simulink model "Accelerator_Pedal_Position_Sensor_APP_Coherency"  (R2022b)
settings: Solver=FixedStepDiscrete  StartTime=0.0  StopTime=10.0  RelTol=1e-3
libraries: simulink x5
settings Model: Creator=yasso  LastModifiedBy=yasso
settings DataIOCC: ExternalInput=[tt, u3, u4]  LoadExternalInput=on

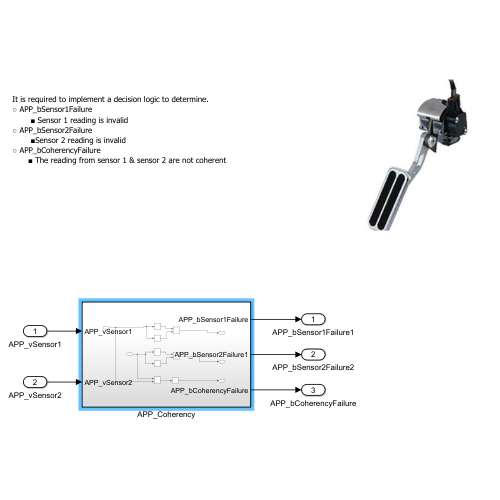
[thumbnail: Simulink's stored preview of the top-level diagram]
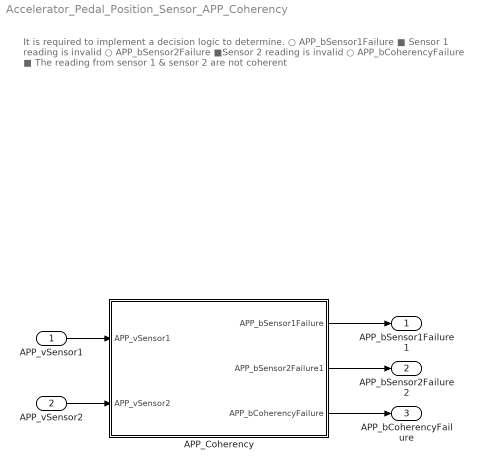
== system Accelerator_Pedal_Position_Sensor_APP_Coherency ==
  note: It is required to implement a decision logic to determine.
      | ○ APP_bSensor1Failure
      | ■ Sensor 1 reading is invalid
      | ○ APP_bSensor2Failure
      | ■Sensor 2 reading is invalid
      | ○ APP_bCoherencyFailure
      | ■ The reading from sensor 1 & sensor 2 are not coherent
  APP_vSensor1 : Inport
  APP_vSensor2 : Inport  Port=2
  APP_Coherency : Subsystem
  APP_bSensor1Failure1 : Outport
  APP_bSensor2Failure2 : Outport  Port=2
  APP_bCoherencyFailure : Outport  Port=3
  wires:
  APP_vSensor1/1 -> APP_Coherency/1(APP_vSensor1)
  APP_Coherency/3(APP_bCoherencyFailure) -> APP_bCoherencyFailure/1
  APP_Coherency/1(APP_bSensor1Failure) -> APP_bSensor1Failure1/1
  APP_Coherency/2(APP_bSensor2Failure1) -> APP_bSensor2Failure2/1
  APP_vSensor2/1 -> APP_Coherency/2(APP_vSensor2)

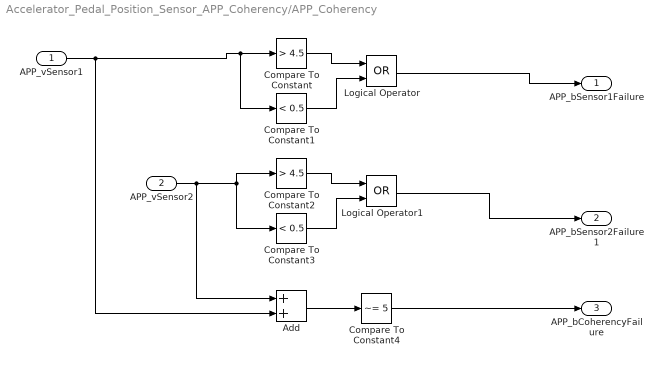
== system Accelerator_Pedal_Position_Sensor_APP_Coherency/APP_Coherency ==
  APP_vSensor1 : Inport
  APP_vSensor2 : Inport  Port=2
  Add : Sum
  Compare To Constant : simulink/Logic and Bit Operations/Compare To Constant  relop=>  const=4.5  OutDataTypeStr=boolean
  Compare To Constant1 : simulink/Logic and Bit Operations/Compare To Constant  relop=<  const=0.5  OutDataTypeStr=boolean
  Compare To Constant2 : simulink/Logic and Bit Operations/Compare To Constant  relop=>  const=4.5  OutDataTypeStr=boolean
  Compare To Constant3 : simulink/Logic and Bit Operations/Compare To Constant  relop=<  const=0.5  OutDataTypeStr=boolean
  Compare To Constant4 : simulink/Logic and Bit Operations/Compare To Constant  relop=~=  const=5  OutDataTypeStr=boolean
  Logical Operator : Logic  Operator=OR  AllPortsSameDT=off  OutDataTypeStr=boolean
  Logical Operator1 : Logic  Operator=OR  AllPortsSameDT=off  OutDataTypeStr=boolean
  APP_bSensor1Failure : Outport
  APP_bSensor2Failure1 : Outport  Port=2
  APP_bCoherencyFailure : Outport  Port=3
  wires:
  APP_vSensor1/1 -> Compare To Constant1/1, Compare To Constant/1, Add/2
  Compare To Constant/1 -> Logical Operator/1
  APP_vSensor2/1 -> Add/1, Compare To Constant3/1, Compare To Constant2/1
  Compare To Constant2/1 -> Logical Operator1/1
  Compare To Constant3/1 -> Logical Operator1/2
  Add/1 -> Compare To Constant4/1
  Compare To Constant4/1 -> APP_bCoherencyFailure/1
  Logical Operator/1 -> APP_bSensor1Failure/1
  Logical Operator1/1 -> APP_bSensor2Failure1/1
  Compare To Constant1/1 -> Logical Operator/2
